simulink model "humanModel"  (R2022b)
settings: Solver=ode1  StartTime=0.0  StopTime=10.0  FixedStep=dt  RelTol=1e-3
values from neighbouring files (symbols this model uses):
  dt = hmn.generalParamSet.dt    [Human.m]    (also in Human_COM.m; Run__holisticModel.m = 0.005; Run__human.m = 0.005; Run__plotFigures.m)
settings Model: Creator=rsharifr  LastModifiedBy=rsharifr

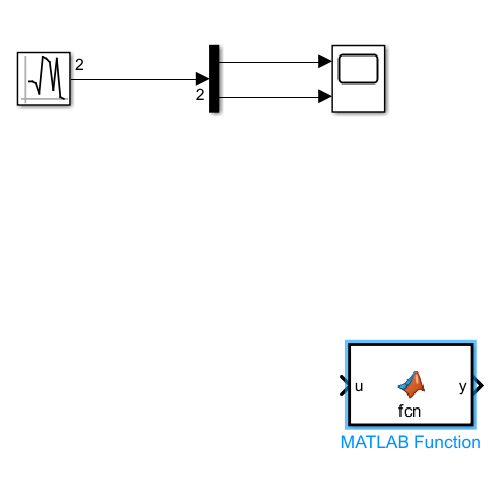
[thumbnail: Simulink's stored preview of the top-level diagram]
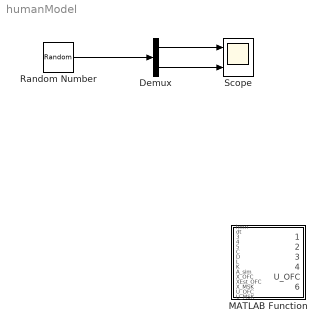
== system humanModel ==
  Demux : Demux  Outputs=2
  MATLAB Function : MATLAB Function  TreatAsAtomicUnit=on
  Random Number : RandomNumber  Mean=[0;0]  Variance=[1;1]  Seed=[0,1]  SampleTime=dt
  Scope : Scope  NumInputPorts=2
  wires:
  Random Number/1 -> Demux/1
  Demux/1 -> Scope/1
  Demux/2 -> Scope/2

== matlab function humanModel/MATLAB Function ==
  data: hmn input; X_OFC_update output; dt input; Omega_omega input; Omega_xi input; Omega_eta input; C input; D input; L input; K input; A_sim input; X_OFC input; XEst_OFC input; X_MSK input; U_OFC input; U_MSK input; XEst_OFC_update output; a_ref_ofc output; XDOT_MSK output; U_OFC output; U_MSK output
function [X_OFC_update, XEst_OFC_update, a_ref_ofc, XDOT_MSK, U_OFC, U_MSK] = ...
    fcn(hmn, dt, ...
    Omega_omega, Omega_xi, Omega_eta, C, D, ...
    L,K, A_sim, ...
    X_OFC, XEst_OFC, X_MSK, U_OFC, U_MSK)

%%%%%% OFC's integral step
sensoryNoise = mvnrnd(zeros(p,1),Omega_omega)';
processNoise = mvnrnd(zeros(n,1),Omega_xi)';
internalNoise = mvnrnd(zeros(n,1),Omega_eta)';

% use this to decouple OFC from MSK. Useful for OFC debugging
%     stateDependentNoise = 0;
%     for isdn = 1:size(D,3)
%         stateDependentNoise = stateDependentNoise + randn*D(:,:,isdn)*X_OFC';
%     end
%     yz = H*hmn.ofcResults.currentX + sensoryNoise + stateDependentNoise;


U_OFC = -L*XEst_OFC;

controlDependentNoise = 0;
for icdn = 1:m
    controlDependentNoise = controlDependentNoise + randn*C(:,:,icdn)*U_OFC;
end

X_OFC_update = A_sim*hmn.ofcResults.currentX + B*hmn.ofcResults.currentU + processNoise + controlDependentNoise;
diff_X_ofc = (X_OFC_update - X_OFC)/dt;

%%%%%%% Generate high-level commands

a_ref_ofc = diff_X_ofc(3:4); % this works better
%     a_ref_ofc = diff_XEst_ofc(3:4);
%                 F_ref_ofc = hmn.ofcResults.currentX(5:6);
%     a_ref_ofc = hmn.ofcResults.currentU;

%%%%%%% MSK's step
q_SH = hmn.getOutputs_msk(hmn.mskResults.currentY).q(1);
q_EL = hmn.getOutputs_msk(hmn.mskResults.currentY).q(2);
qdot_SH = hmn.getOutputs_msk(hmn.mskResults.currentY).qdot(1);
qdot_EL = hmn.getOutputs_msk(hmn.mskResults.currentY).qdot(2);

Fpert_est = hmn.ofcResults.currentXEst(7:8);

syn = interpn(1:Nmuscle,1:NoSyn,thetaSHset,thetaELset,  synergySet  ,1:Nmuscle,1:NoSyn,q_SH,q_EL);
[basis_acc,basis_F] = calcBasis(syn, q_SH,q_EL,armDamping);

a_ref_tilde = hmn.CorrectAccRef(a_ref_ofc,q_SH,q_EL,qdot_SH,qdot_EL,Fpert_est);

coeff = lsqnonneg(basis_acc,a_ref_tilde);
% coeff = lsqnonneg(basis_F,F_ref_ofc);
hmn.mskResults.currentU = syn*coeff;
hmn.mskResults.currentU = min(1,max(0,hmn.mskResults.currentU));
hmn.mskResults.currentU = hmn.mskResults.currentU .* (1+0.02*randn(size(hmn.mskResults.currentU)));


[hmn.mskResults.currentXdot, ~, hmn.mskResults.currentY] = PlanarArm(0,hmn.mskResults.currentX,[Fpert(2);Fpert(1);hmn.mskResults.currentU],armDamping);

hmn.mskResults.Udata(i,:) = hmn.mskResults.currentU';
hmn.mskResults.Ydata(i,:) = hmn.mskResults.currentY';
hmn.mskResults.Xdata(i,:) = hmn.mskResults.currentX';
hmn.mskResults.currentX = hmn.mskResults.currentX + hmn.mskResults.currentXdot * dt;

%%%%%%% Estimator's integration step
handPos = hmn.getOutputs_msk(hmn.mskResults.currentY).hand_p - hmn.generalParamSet.targetPos_abs;
handVel = hmn.getOutputs_msk(hmn.mskResults.currentY).hand_v;

stateDependentNoise = 0;
for isdn = 1:size(D,3)
    stateDependentNoise = stateDependentNoise + randn*D(:,:,isdn)*hmn.ofcResults.currentX;
end
yz = [handPos; handVel; hmn.ofcResults.currentX(5:6); Fpert] + sensoryNoise + stateDependentNoise;

newXEst_ofc = A(:,:,i)*hmn.ofcResults.currentXEst + B*hmn.ofcResults.currentU + K(:,:,i)*(yz-H*hmn.ofcResults.currentXEst) + internalNoise;
diff_XEst_ofc = (newXEst_ofc - hmn.ofcResults.currentXEst)/dt;
hmn.ofcResults.XEstdata(i,:) = hmn.ofcResults.currentXEst';
hmn.ofcResults.currentXEst = newXEst_ofc; %TODO check i or i+1, both here and above

%%%%%%% plot this arm path
if plotResults && mod(i,10)==1
    cmap = copper(nStep);
    [hnd, elb] = hmn.getHandPosition(q_SH,q_EL);
    plot([0,elb(1),hnd(1)], [0,elb(2),hnd(2)],'-o','LineWidth',2,'Color',cmap(i,:))
    scatter(hmn.ofcResults.currentX(1)+hmn.generalParamSet.targetPos_abs(1), hmn.ofcResults.currentX(2)+hmn.generalParamSet.targetPos_abs(2),'s','filled')
    scatter(hmn.ofcResults.currentXEst(1)+hmn.generalParamSet.targetPos_abs(1), hmn.ofcResults.currentXEst(2)+hmn.generalParamSet.targetPos_abs(2),100,'x','MarkerEdgeColor','r','LineWidth',2)
end

end
